simulink model "block_dob"  (R2019b)
settings: Solver=FixedStepAuto  StartTime=0.0  StopTime=1  FixedStep=H  RelTol=1e-3
values from neighbouring files (symbols this model uses):
  H = 1000e-6    (= 0.001)    [script_DOB.m]
  Pn = 1.8/(0.005*s^2 + 0.032*s)    [script_DOB.m]
  Q = w^2/(s^2 + 2*w*s + w^2)    [script_DOB.m]
libraries: cstblocks x4, simulink x1
settings Model: Creator=Wataru  LastModifiedBy=ltfsm
settings SFSimCC: CustomCodeUndefinedFunction=UseInterfaceOnly

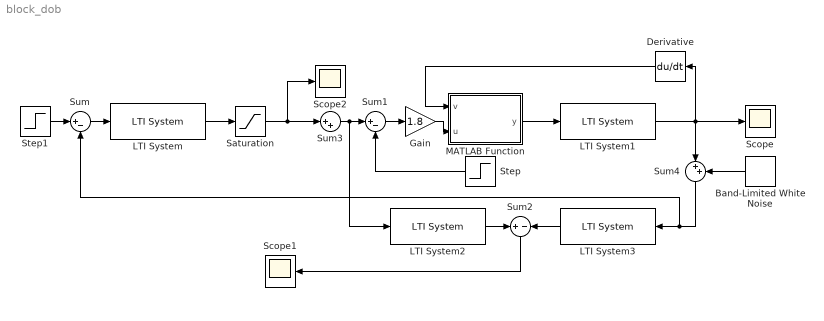
== system block_dob ==
  Band-Limited White Noise : simulink/Sources/Band-Limited White Noise  Cov=1e-7  Ts=H  seed=[2341]
  Derivative : Derivative
  Gain : Gain  Gain=1.8
  LTI System : cstblocks/LTI System  sys=Cpd  IC=[]
  LTI System1 : cstblocks/LTI System  sys=P  IC=[]
  LTI System2 : cstblocks/LTI System  sys=Q  IC=[]
  LTI System3 : cstblocks/LTI System  sys=Q/Pn  IC=[]
  MATLAB Function : MATLAB Function  TreatAsAtomicUnit=on
  Saturation : Saturate  UpperLimit=5  LowerLimit=-5
  Scope : Scope
  Scope1 : Scope
  Scope2 : Scope
  Step : Step  Time=0.6  After=0  SampleTime=0
  Step1 : Step  Time=0.2  After=2  SampleTime=0
  Sum : Sum  Inputs=|+-
  Sum1 : Sum  Inputs=|+-
  Sum2 : Sum  Inputs=+|-
  Sum3 : Sum  Inputs=|++
  Sum4 : Sum  Inputs=|++
  wires:
  Step1/1 -> Sum/1
  Sum/1 -> LTI System/1
  Step/1 -> Sum1/2
  LTI System1/1 -> Sum4/1, Scope/1, Derivative/1
  LTI System2/1 -> Sum2/1
  LTI System3/1 -> Sum2/2
  LTI System/1 -> Saturation/1
  Sum3/1 -> Sum1/1, LTI System2/1
  Sum2/1 -> Scope1/1
  Sum4/1 -> Sum/2, LTI System3/1
  Band-Limited White Noise/1 -> Sum4/2
  MATLAB Function/1(y) -> LTI System1/1
  Derivative/1 -> MATLAB Function/1(v)
  Sum1/1 -> Gain/1
  Gain/1 -> MATLAB Function/2(u)
  Saturation/1 -> Scope2/1, Sum3/1

== matlab function block_dob/MATLAB Function ==
  data: v input; u input; y output
function y = fcn(v, u)
Ns = 0.1;
Nd = 0.05;

    if v == 0
        y = abs(u)-Ns;
        if y < 0
            y = 0;
        else
            y = sign(y)*y;
        end
    else 
        y = abs(u)-sign(u*v)*Nd;
        y = sign(u)*y;
    end
